simulink model "sumadorproducto"  (R2014a)
settings: Solver=ode45  StartTime=0.0  StopTime=10.0  RelTol=1e-3
settings Model: Creator=nigrobyte  LastModifiedBy=nigrobyte

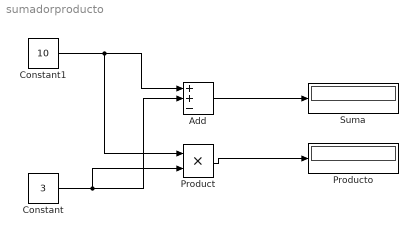
== system sumadorproducto ==
  Add : Sum  Inputs=++-
  Constant : Constant  Value=3
  Constant1 : Constant  Value=10
  "Product " : Product  Inputs=**
  "Producto " : Display
  Suma : Display
  wires:
  Constant1/1 -> "Product "/1, Add/1
  Add/1 -> Suma/1
  Constant/1 -> "Product "/2, Add/2
  "Product "/1 -> "Producto "/1
